simulink subsystem "Subsystem"  (R2022a)
settings: Solver=VariableStepAuto  StartTime=0.0  StopTime=10.0  RelTol=1e-3
settings Model: Creator=ssen  LastModifiedBy=ssen
settings SolverCC: MaxZcPerStep=1

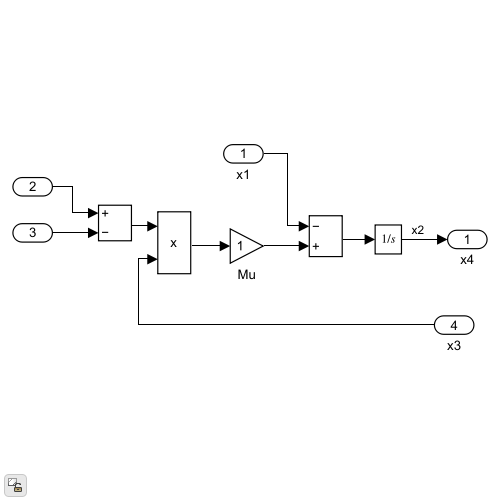
[thumbnail: Simulink's stored preview of the top-level diagram]
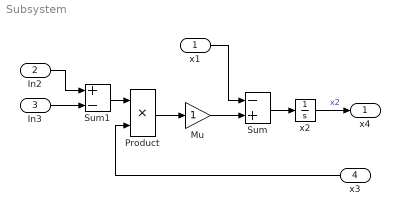
== system Subsystem ==
  x1 : Inport
  In2 : Inport  Port=2
  In3 : Inport  Port=3
  x3 : Inport  Port=4
  Mu : Gain  SaturateOnIntegerOverflow=on  OutDataTypeStr=Inherit: Same as input  ParamDataTypeStr=Inherit: Same as input
  Product : Product  InputSameDT=on  RndMeth=Zero  SaturateOnIntegerOverflow=on  OutDataTypeStr=Inherit: Same as first input
  Sum : Sum  Inputs=-+  InputSameDT=on  SaturateOnIntegerOverflow=on  OutDataTypeStr=Inherit: Same as first input
  Sum1 : Sum  Inputs=+-  InputSameDT=on  SaturateOnIntegerOverflow=on  OutDataTypeStr=Inherit: Same as first input
  x2 : Integrator
  x4 : Outport
  wires:
  Product/1 -> Mu/1
  x3/1 -> Product/2
  Sum/1 -> x2/1
  x1/1 -> Sum/1
  Sum1/1 -> Product/1
  Mu/1 -> Sum/2
  In2/1 -> Sum1/1
  x2/1 -> x4/1  "x2"
  In3/1 -> Sum1/2
